simulink model "torqueBalancingR2015bS86"  (Simulink 8.6)
settings: Solver=FixedStepDiscrete  StartTime=0.0  StopTime="CONFIG.SIMULATION_TIME "  FixedStep=CONFIG.Ts  RelTol=1e-3
InitFcn:
  | cd(fileparts(which(bdroot)));
  | initTorqueBalancing;
values from neighbouring files (symbols this model uses):
  WBT_modelName = 'matlabTorqueBalancing'    [initTorqueBalancing.m]    (also in initTorqueBalancingPC.m)
undefined symbols (not defined in the file or in its folder): bVectorConstraints, CONFIG, ConstraintsMatrix, DiscIntNeverNeededParam, gain, references, reg, ROBOT_DOF, ROBOT_DOF_FOR_SIMULINK, sat, SM, sm, WBT_robotName
libraries: WBToolboxLibrary x118, simulink x11
(part 3 of 3)

== matlab function DesValues/State Machine/nu/MATLAB Function ==
  data: JcLeftFoot input double; JcRightFoot input double; activeFeetConstraints input double; y output double; qD input double; reg parameter double
function y = fcn(JcLeftFoot,JcRightFoot,activeFeetConstraints,qD,reg)
%#codegen

Jc = [activeFeetConstraints(1)*JcLeftFoot;
      activeFeetConstraints(2)*JcRightFoot];

pinvJb = pinvDamped(Jc(:,1:6),reg.pinvDampVb);  
  
% pinvJb = pinv(Jc(:,1:6));

y = -pinvJb*Jc(:,7:end)*qD;

== matlab function DesValues/State Machine/stateMachineFCN ==
  data: wrench_rightFoot input double; wrench_leftFoot input double; w_H_b output double; CoMDes output double; qDes output double; constraints output double; CoM_0 input double; q0 input double; l_sole_CoM input double; r_sole_CoM input double; qj input double; t input double; l_sole_H_b input double; r_sole_H_b input double; sm parameter double; impedances output double; kpCom output double; kdCom output double; gain parameter double; currentState output double; jointsSmoothingTime output double
function [w_H_b, CoMDes,qDes,constraints,impedances,kpCom,kdCom,currentState,jointsSmoothingTime] = ...
    stateMachineFCN(wrench_rightFoot,wrench_leftFoot,CoM_0, q0, l_sole_CoM,r_sole_CoM,qj, t, l_sole_H_b, r_sole_H_b, sm,gain)
%#codegen
 
[w_H_b, CoMDes,qDes,constraints,impedances,kpCom,kdCom,currentState,jointsSmoothingTime] = ...
    stateMachine(CoM_0, q0, l_sole_CoM,r_sole_CoM,qj, t, wrench_rightFoot,wrench_leftFoot,l_sole_H_b, r_sole_H_b, sm,gain);

== matlab function DesValues/State Machine Walking/w_H_root_link1/fromImuToHomogeousTransformFCN ==
  data: imu_H_link input double; imu_H_link_0 input double; link_H_root input double; inertial_0 input double; inertial input double; neck input double; w_H_root output double; CONFIG parameter double
function w_H_root = fromBaseToWorldWithImuFCN(imu_H_link,imu_H_link_0,link_H_root,inertial_0,inertial,neck,CONFIG)
%#codegen
w_H_root = fromBaseToWorldWithImu(imu_H_link,imu_H_link_0,link_H_root,inertial_0,inertial,neck,CONFIG);

== matlab function Dump and visualize/plotNorms/norm ==
  data: u input double; normU output double
function normU = fcn(u)
%#codegen

normU = norm(u);

== matlab function Dump and visualize/plotNorms/norm1 ==
  data: u input double; normU output double
function normU = fcn(u)
%#codegen

normU = norm(u);

== matlab function controller_QP/tau(f)  ==
  data: tauModel output double; Sigma output double; NA output double; fHdotDesC1C2 output double; HessianMatrixQP1Foot output double; gradientQP1Foot output double; ConstraintsMatrixQP1Foot output double; bVectorConstraintsQp1Foot output double; HessianMatrixQP2Feet output double; gradientQP2Feet output double; ConstraintsMatrixQP2Feet output double; bVectorConstraintsQp2Feet output double; constraints input double; ROBOT_DOF_FOR_SIMULINK input double; ConstraintsMatrix input double; bVectorConstraints input double; q input double; qDes input double; v input double; M input double; h input double; H input double; intHw input double; w_H_l_sole input double; w_H_r_sole input double; JL input double; JR input double; dJLv input double; dJRv input double; xcom input double; J_CoM input double; desired_x_dx_ddx_CoM input double; gainsPCOM input double; gainsDCOM input double; impedances input double; intErrorCoM input double; ki_int_qtilde input double; reg parameter double; gain parameter double; errorCoM output double; qTilde output double; f output double
function [tauModel,Sigma,NA,fHdotDesC1C2, ...
          HessianMatrixQP1Foot,gradientQP1Foot,ConstraintsMatrixQP1Foot,bVectorConstraintsQp1Foot,...
          HessianMatrixQP2Feet,gradientQP2Feet,ConstraintsMatrixQP2Feet,bVectorConstraintsQp2Feet,...
          errorCoM,qTilde,f]    =  ...
          balancingControllerFCN(constraints,ROBOT_DOF_FOR_SIMULINK,ConstraintsMatrix,bVectorConstraints,...
          q,qDes,v, M, h , H,intHw,w_H_l_sole, w_H_r_sole, JL,JR, dJLv,dJRv, xcom,J_CoM, desired_x_dx_ddx_CoM,...
          gainsPCOM,gainsDCOM,impedances, intErrorCoM,ki_int_qtilde,reg,gain)
%#codegen
    [tauModel,Sigma,NA,fHdotDesC1C2, ...
                  HessianMatrixQP1Foot,gradientQP1Foot,ConstraintsMatrixQP1Foot,bVectorConstraintsQp1Foot,...
                  HessianMatrixQP2Feet,gradientQP2Feet,ConstraintsMatrixQP2Feet,bVectorConstraintsQp2Feet,...
                  errorCoM,qTilde,f]    =  ...
                  balancingController(constraints,ROBOT_DOF_FOR_SIMULINK,ConstraintsMatrix,bVectorConstraints,...
                  q,qDes,v, M, h , H,intHw,w_H_l_sole, w_H_r_sole, JL,JR, dJLv,dJRv, xcom,J_CoM, desired_x_dx_ddx_CoM,...
                  gainsPCOM,gainsDCOM,impedances,intErrorCoM,ki_int_qtilde,reg,gain);
end

== matlab function emergency stop: joint limits/MATLAB Function ==
  data: umin input double; umax input double; u input double; inRange output double; tol input double
function inRange = checkRange(umin, umax, u, tol)
%#codegen

res = u < umin + tol | u > umax - tol;
res = sum(res);
if res==0
    inRange = 1;
else
    inRange = 0;
    u < umin + tol | u > umax - tol
end

== matlab function controller_QP/integralOf Hw1/MATLAB Function ==
  data: qjErr input double; JL input double; JR input double; vbEquivalent output double; reg parameter double; activeFeetConstraints input double
 function vbEquivalent = generateReferencesForH(qjErr,JL,JR,reg,activeFeetConstraints)
%#codegen
if activeFeetConstraints(1) == 1
    
pinvJb             = (JL(:,1:6)'*JL(:,1:6) + reg.pinvDampVb*eye(6))\JL(:,1:6)';
vbEquivalent       = -pinvJb*JL(:,7:end)*qjErr;
else
    
pinvJb             = (JR(:,1:6)'*JR(:,1:6) + reg.pinvDampVb*eye(6))\JR(:,1:6)';
vbEquivalent       = -pinvJb*JR(:,7:end)*qjErr;
end
    
end

== matlab function DesValues/State Machine/visualise inertial/Visualize hom transf1/MATLAB Function ==
  data: R input double; rollPitchYaw output double
function rollPitchYaw = buildHomogenousTranformation(R)
%#codegen

rollPitchYaw = rollPitchYawFromRotation(R);

rollPitchYaw = rollPitchYaw*180/pi;

== matlab function DesValues/State Machine/visualise inertial/Visualize hom transf2/MATLAB Function ==
  data: R input double; rollPitchYaw output double
function rollPitchYaw = buildHomogenousTranformation(R)
%#codegen

rollPitchYaw = rollPitchYawFromRotation(R);

rollPitchYaw = rollPitchYaw*180/pi;

== matlab function DesValues/State Machine/visualise inertial/Visualize hom transf4/MATLAB Function ==
  data: R input double; rollPitchYaw output double
function rollPitchYaw = buildHomogenousTranformation(R)
%#codegen

rollPitchYaw = rollPitchYawFromRotation(R);

rollPitchYaw = rollPitchYaw*180/pi;

== matlab function DesValues/State Machine/visualise inertial/Visualize hom transf5/MATLAB Function ==
  data: R input double; rollPitchYaw output double
function rollPitchYaw = buildHomogenousTranformation(R)
%#codegen

rollPitchYaw = rollPitchYawFromRotation(R);

rollPitchYaw = rollPitchYaw*180/pi;

== matlab function DesValues/State Machine/visualise inertial/Visualize hom transf6/MATLAB Function ==
  data: R input double; rollPitchYaw output double
function rollPitchYaw = buildHomogenousTranformation(R)
%#codegen

rollPitchYaw = rollPitchYawFromRotation(R);

rollPitchYaw = rollPitchYaw*180/pi;

== matlab function DesValues/State Machine/visualise inertial/Visualize hom transf3/MATLAB Function ==
  data: R input double; rollPitchYaw output double
function rollPitchYaw = buildHomogenousTranformation(R)
%#codegen

rollPitchYaw = rollPitchYawFromRotation(R);

rollPitchYaw = rollPitchYaw*180/pi;

== matlab function DesValues/State Machine/visualise inertial/w_H_root_link4/fromImuToHomogeousTransformFCN ==
  data: imu_H_link input double; imu_H_link_0 input double; link_H_root input double; inertial_0 input double; inertial input double; neck input double; w_H_root output double; CONFIG parameter double
function w_H_root = fromBaseToWorldWithImuFCN(imu_H_link,imu_H_link_0,link_H_root,inertial_0,inertial,neck,CONFIG)
%#codegen
w_H_root = fromBaseToWorldWithImu(imu_H_link,imu_H_link_0,link_H_root,inertial_0,inertial,neck,CONFIG);

== matlab function controller_QP/integralOf Hw1/w_H_root_link4/fromImuToHomogeousTransformFCN ==
  data: imu_H_link input double; imu_H_link_0 input double; link_H_root input double; inertial_0 input double; inertial input double; neck input double; w_H_root output double; CONFIG parameter double
function w_H_root = fromBaseToWorldWithImuFCN(imu_H_link,imu_H_link_0,link_H_root,inertial_0,inertial,neck,CONFIG)
%#codegen
w_H_root = fromBaseToWorldWithImu(imu_H_link,imu_H_link_0,link_H_root,inertial_0,inertial,neck,CONFIG);
